simulink model "simulink51"  (R2020a)
settings: Solver=VariableStepAuto  StartTime=0.0  StopTime=10.0  RelTol=1e-3
settings Model: Creator=16002  LastModifiedBy=16002

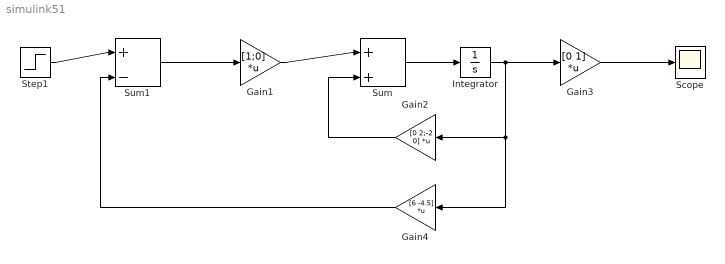
== system simulink51 ==
  Gain1 : Gain  Gain=[1;0]  Multiplication=Matrix(K*u)
  Gain2 : Gain  Gain=[0 2;-2 0]  Multiplication=Matrix(K*u)
  Gain3 : Gain  Gain=[0 1]  Multiplication=Matrix(K*u)
  Gain4 : Gain  Gain=[6 -4.5]  Multiplication=Matrix(K*u)
  Integrator : Integrator
  Scope : Scope
  Step1 : Step  SampleTime=0
  Sum : Sum  Inputs=|++
  Sum1 : Sum  Inputs=|+-
  wires:
  Gain1/1 -> Sum/1
  Gain2/1 -> Sum/2
  Sum/1 -> Integrator/1
  Integrator/1 -> Gain4/1, Gain2/1, Gain3/1
  Gain3/1 -> Scope/1
  Gain4/1 -> Sum1/2
  Sum1/1 -> Gain1/1
  Step1/1 -> Sum1/1
